simulink subsystem "Vorsteuerung_Fa_avRegler"  (R2020a)
settings: Solver=VariableStepAuto  StartTime=0.0  StopTime=10.0  RelTol=1e-3
model mask{K_p_v=0, a_max=0, vorst_c=on, vorst_d=on}
  mask prompts: K_p_v "a/v-Regler Kpv"; a_max "Soll-Beschleunigung Max (AW)"; vorst_c "Vorsteuerung Coulomb Reibung"; vorst_d "Vorsteuerung Viskose Reibung"
settings Model: Creator=Tobias  LastModifiedBy=Tobias

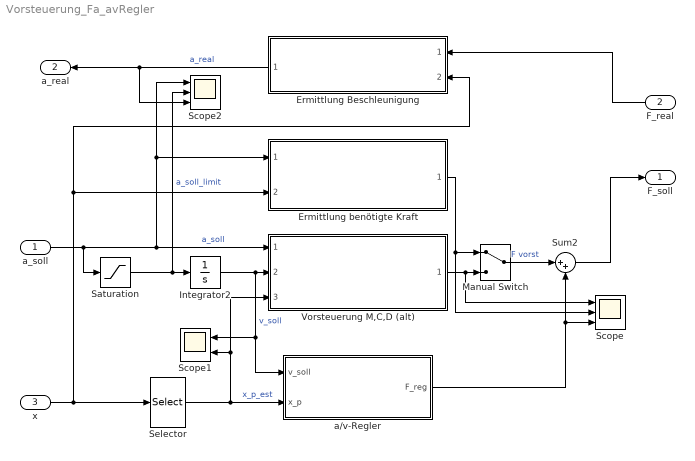
== system Vorsteuerung_Fa_avRegler ==
  a_soll : Inport
  F_real : Inport  Port=2
  x : Inport  Port=3
  Ermittlung Beschleunigung : Subsystem  ReferencedSubsystem=SchlittenGleichungBeschleunigung
  Ermittlung benötigte Kraft : Subsystem  ReferencedSubsystem=SchlittenGleichungKraft
  Integrator2 : Integrator
  Manual Switch : ManualSwitch
  Saturation : Saturate  UpperLimit=a_max  LowerLimit=-a_max
  Scope : Scope  NumInputPorts=3
  Scope1 : Scope  NumInputPorts=2
  Scope2 : Scope  NumInputPorts=3
  Selector : Selector  InputPortWidth=6  IndexOptions=Index vector (dialog)  Indices=[2]  OutputSizes=1
  Sum2 : Sum  Inputs=|++
  Vorsteuerung M,C,D (alt) : Subsystem  ReferencedSubsystem=SchlittenVorsteuerung  SP=simparams.gesamtmodell.schlittenpendel  vorst=simparams.vorst
  a/v-Regler : Subsystem
  F_soll : Outport
  a_real : Outport  Port=2
  wires:
  Selector/1 -> Scope1/2, Vorsteuerung M,C,D (alt)/3, a/v-Regler/2(x_p)  "x_p_est"
  Integrator2/1 -> a/v-Regler/1(v_soll), Scope1/1, Vorsteuerung M,C,D (alt)/2  "v_soll"
  a_soll/1 -> Saturation/1, Scope2/1, Ermittlung benötigte Kraft/1, Vorsteuerung M,C,D (alt)/1  "a_soll"
  Sum2/1 -> F_soll/1
  Manual Switch/1 -> Sum2/1  "F vorst"
  x/1 -> Ermittlung Beschleunigung/2, Ermittlung benötigte Kraft/2, Selector/1
  a/v-Regler/1(F_reg) -> Sum2/2, Scope/3
  F_real/1 -> Ermittlung Beschleunigung/1
  Ermittlung Beschleunigung/1 -> a_real/1, Scope2/3  "a_real"
  Ermittlung benötigte Kraft/1 -> Scope/2, Manual Switch/1
  Vorsteuerung M,C,D (alt)/1 -> Manual Switch/2, Scope/1
  Saturation/1 -> Integrator2/1, Scope2/2  "a_soll_limit"

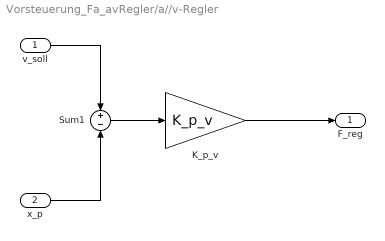
== system Vorsteuerung_Fa_avRegler/a//v-Regler ==
  v_soll : Inport
  x_p : Inport  Port=2
  K_p_v : Gain  Gain=K_p_v
  Sum1 : Sum  Inputs=+|-
  F_reg : Outport
  wires:
  Sum1/1 -> K_p_v/1
  x_p/1 -> Sum1/2
  v_soll/1 -> Sum1/1
  K_p_v/1 -> F_reg/1
